simulink model "dc_motor_pi_control"  (R2025b)
settings: Solver=VariableStepAuto  StartTime=0.0  StopTime=10.0  RelTol=1e-3
settings Model: Creator=imman  LastModifiedBy=imman

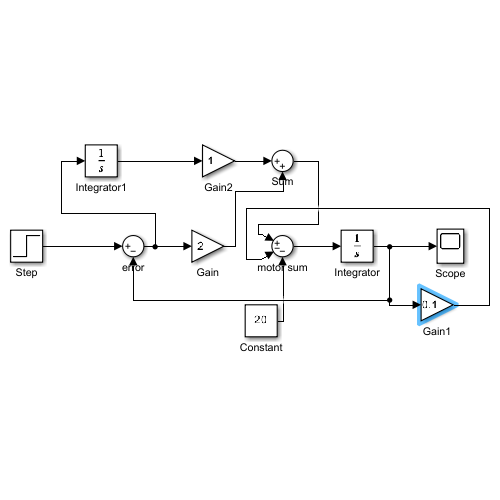
[thumbnail: Simulink's stored preview of the top-level diagram]
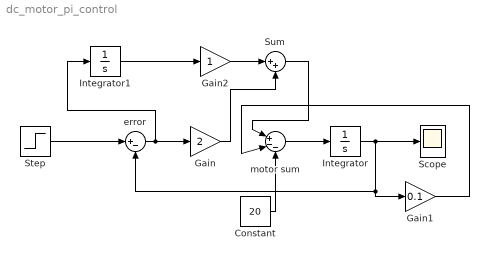
== system dc_motor_pi_control ==
  Constant : Constant  Value=20
  Gain : Gain  Gain=2
  Gain1 : Gain  Gain=0.1
  Gain2 : Gain
  Integrator : Integrator
  Integrator1 : Integrator
  Scope : Scope
      settings: ActiveDisplayYMinimum=-86.793062938916776  ActiveDisplayYMaximum=135.94924182909529
  Step : Step  Time=0  After=100  SampleTime=0
  Sum : Sum  Inputs=|++
  error : Sum  Inputs=|+-
  motor sum : Sum  Inputs=|+--
  wires:
  Step/1 -> error/1
  error/1 -> Integrator1/1, Gain/1
  Integrator/1 -> Scope/1, error/2, Gain1/1
  Gain1/1 -> motor sum/2
  Gain/1 -> Sum/2
  motor sum/1 -> Integrator/1
  Constant/1 -> motor sum/3
  Integrator1/1 -> Gain2/1
  Gain2/1 -> Sum/1
  Sum/1 -> motor sum/1
